simulink model "Signal_Builder_verif"  (Simulink 8.4)
settings: Solver=ode45  StartTime=0.0  StopTime=10.0  RelTol=1e-3
undefined symbols (not defined in the file): sigbuilder_block
settings Model: Creator=Romain  LastModifiedBy=hbourbou
settings DataIOCC: SignalLoggingSaveFormat=Dataset
settings OptimizationCC: ExpressionDepthLimit=128
settings DebuggingCC: SolverPrmCheckMsg=none  FcnCallInpInsideContextMsg=EnableAllAsError  FrameProcessingCompatibilityMsg=error  StateNameClashWarn=none
settings GRTTargetCC: CombineOutputUpdateFcns=on  GRTInterface=off

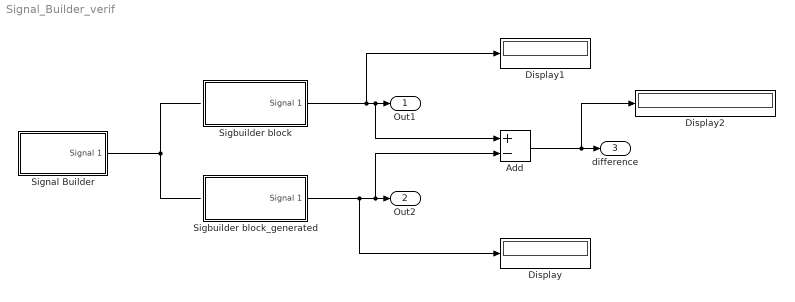
== system Signal_Builder_verif ==
  Add : Sum  Inputs=+-
  Display : Display
  Display1 : Display
  Display2 : Display
  Sigbuilder block : Subsystem  Tag=STV Subsys  LoadFcn=sigbuilder_block('load');  StartFcn=sigbuilder_block('start');  StopFcn=sigbuilder_block('stop');  ClipboardFcn=sigbuilder_block('clipboard');  mask(Sigbuilder block){}
      mask help: Simulink:masks:SigbuilderBlock_MD
      mask init:
      | if ~strcmp(get_param(bdroot(gcbh),'SimulationStatus'),'stopped') tuvar = sigbuilder_block('maskInit'); end
      settings: CopyFcn=sigbuilder_block('copy');  DeleteFcn=sigbuilder_block('delete');  ModelCloseFcn=sigbuilder_block('modelClose');  PreSaveFcn=sigbuilder_block('preSave');  PauseFcn=sigbuilder_block('pause');  ContinueFcn=sigbuilder_block('continue');  NameChangeFcn=sigbuilder_block('namechange');  OpenFcn=sigbuilder_block('open',[437.6 199.2 550.4 400 ]);  CloseFcn=sigbuilder_block('close');
      mask Display: plot(0, 0, 100, 100,[2, 2, 32, 32, 2], [68, 8, 8, 68, 68],[32, 2], [38, 38], [32, 19, 2],[53, 60, 44], [32, 17, 17, 2],[16, 16, 31, 31]);txt = getActiveGroup(gcbh);text(2, 100, txt,'verticalAlignment', 'top');
  Sigbuilder block_generated : Subsystem  TreatAsAtomicUnit=on
  Signal Builder : Subsystem  Tag=STV Subsys  LoadFcn=sigbuilder_block('load');  StartFcn=sigbuilder_block('start');  StopFcn=sigbuilder_block('stop');  ClipboardFcn=sigbuilder_block('clipboard');  mask(Sigbuilder block){}
      mask help: Simulink:masks:SigbuilderBlock_MD
      mask init:
      | if ~strcmp(get_param(bdroot(gcbh),'SimulationStatus'),'stopped') tuvar = sigbuilder_block('maskInit'); end
      settings: CopyFcn=sigbuilder_block('copy');  DeleteFcn=sigbuilder_block('delete');  ModelCloseFcn=sigbuilder_block('modelClose');  PreSaveFcn=sigbuilder_block('preSave');  PauseFcn=sigbuilder_block('pause');  ContinueFcn=sigbuilder_block('continue');  NameChangeFcn=sigbuilder_block('namechange');  OpenFcn=sigbuilder_block('open',[437.6 199.2 550.4 400 ]);  CloseFcn=sigbuilder_block('close');
      mask Display: plot(0, 0, 100, 100,[2, 2, 32, 32, 2], [68, 8, 8, 68, 68],[32, 2], [38, 38], [32, 19, 2],[53, 60, 44], [32, 17, 17, 2],[16, 16, 31, 31]);txt = getActiveGroup(gcbh);text(2, 100, txt,'verticalAlignment', 'top');
  Out1 : Outport
  Out2 : Outport  Port=2
  difference : Outport  Port=3
  wires:
  Signal Builder/1(Signal 1) -> ?
  Sigbuilder block/1(Signal 1) -> Display1/1, Add/1, Out1/1
  Sigbuilder block_generated/1(Signal 1) -> Display/1, Add/2, Out2/1
  Add/1 -> Display2/1, difference/1

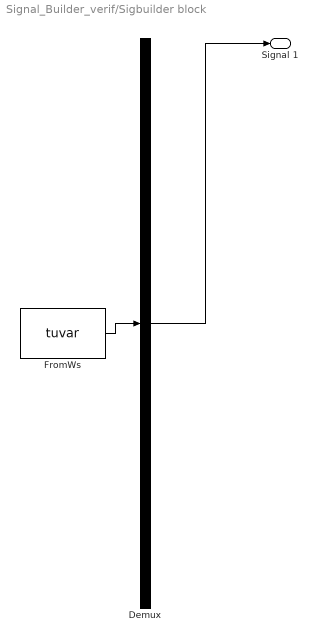
== system Signal_Builder_verif/Sigbuilder block ==
  Demux : Demux  Tag=STV Demux  Outputs=1
  FromWs : FromWorkspace  Tag=STV FromWs  VariableName=tuvar  SampleTime=0  SigBuilderData=DataTag0  VnvData=DataTag1
      SigBuilderData=|
      | common.afterFinalStr = 'Extrapolate'
      | common.sampleTime = 0
      | dataSet.timeRange = [0 10]
      | dataSet.name = 'Group 1'
      | sbobj.Groups.Name = 'Group 1'
      | sbobj.Groups.Signals.Name = 'Signal 1'
      | sbobj.Groups.Signals.XData = [0 4 4 6 6 10]
      | sbobj.Groups.Signals.YData = [0 0.99 1 0.01 0 0]
  Signal 1 : Outport  Tag=STV Outport
  wires:
  FromWs/1 -> Demux/1
  Demux/1 -> Signal 1/1

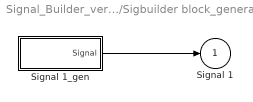
== system Signal_Builder_verif/Sigbuilder block_generated ==
  Signal 1_gen : Subsystem  TreatAsAtomicUnit=on
  Signal 1 : Outport
  wires:
  Signal 1_gen/1(Signal) -> Signal 1/1

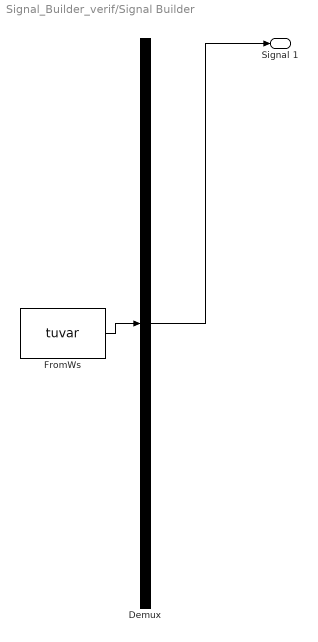
== system Signal_Builder_verif/Signal Builder ==
  Demux : Demux  Tag=STV Demux  Outputs=1
  FromWs : FromWorkspace  Tag=STV FromWs  VariableName=tuvar  SampleTime=0  SigBuilderData=DataTag2  VnvData=DataTag3
      SigBuilderData=|
      | common.afterFinalStr = 'Extrapolate'
      | common.sampleTime = 0
      | dataSet.timeRange = [0 10]
      | dataSet.name = 'Group 1'
      | sbobj.Groups.Name = 'Group 1'
      | sbobj.Groups.Signals.Name = 'Signal 1'
      | sbobj.Groups.Signals.XData = [0 4 4 6 6 10]
      | sbobj.Groups.Signals.YData = [0 0.99 1 0.3 0.26 0]
  Signal 1 : Outport  Tag=STV Outport
  wires:
  Demux/1 -> Signal 1/1
  FromWs/1 -> Demux/1

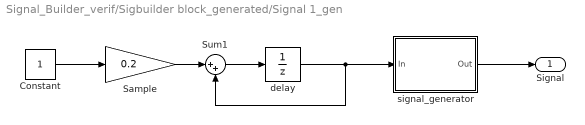
== system Signal_Builder_verif/Sigbuilder block_generated/Signal 1_gen ==
  Constant : Constant
  Sample : Gain  Gain=0.2
  Sum1 : Sum  RequirementInfo={} %GIDa_4fd8ee4a_06a5_4376_942d_ced6baffe973  Inputs=|++
  delay : UnitDelay  SampleTime=-1
  signal_generator : Subsystem  TreatAsAtomicUnit=on
  Signal : Outport  RequirementInfo={} %GIDa_242d5b11_f303_43fe_914a_b04d41914e6e
  wires:
  Sample/1 -> Sum1/1
  Sum1/1 -> delay/1
  Constant/1 -> Sample/1
  delay/1 -> Sum1/2, signal_generator/1(In)
  signal_generator/1(Out) -> Signal/1

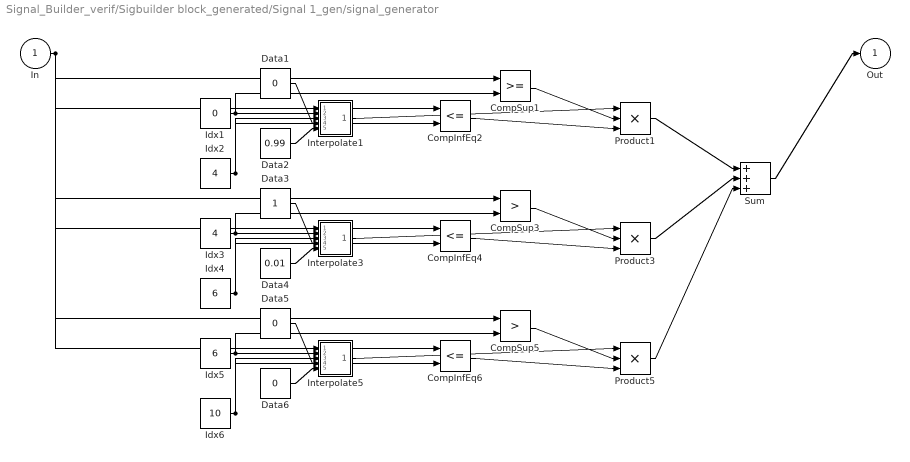
== system Signal_Builder_verif/Sigbuilder block_generated/Signal 1_gen/signal_generator ==
  In : Inport
  CompInfEq2 : RelationalOperator  Operator=<=  InputSameDT=on
  CompInfEq4 : RelationalOperator  Operator=<=  InputSameDT=on
  CompInfEq6 : RelationalOperator  Operator=<=  InputSameDT=on
  CompSup1 : RelationalOperator  InputSameDT=on
  CompSup3 : RelationalOperator  Operator=>  InputSameDT=on
  CompSup5 : RelationalOperator  Operator=>  InputSameDT=on
  Data1 : Constant  Value=0
  Data2 : Constant  Value=0.99
  Data3 : Constant
  Data4 : Constant  Value=0.01
  Data5 : Constant  Value=0
  Data6 : Constant  Value=0
  Idx1 : Constant  Value=0
  Idx2 : Constant  Value=4
  Idx3 : Constant  Value=4
  Idx4 : Constant  Value=6
  Idx5 : Constant  Value=6
  Idx6 : Constant  Value=10
  Interpolate1 : Subsystem  TreatAsAtomicUnit=on
  Interpolate3 : Subsystem  TreatAsAtomicUnit=on
  Interpolate5 : Subsystem  TreatAsAtomicUnit=on
  Product1 : Product  Inputs=***  SaturateOnIntegerOverflow=on  RndMeth=Zero  OutDataTypeStr=Inherit: Same as first input
  Product3 : Product  Inputs=***  SaturateOnIntegerOverflow=on  RndMeth=Zero  OutDataTypeStr=Inherit: Same as first input
  Product5 : Product  Inputs=***  SaturateOnIntegerOverflow=on  RndMeth=Zero  OutDataTypeStr=Inherit: Same as first input
  Sum : Sum  Inputs=+++  SaturateOnIntegerOverflow=on  InputSameDT=on  OutDataTypeStr=Inherit: Same as first input
  Out : Outport
  wires:
  Sum/1 -> Out/1
  Data6/1 -> Interpolate5/5(InportData2)
  Idx6/1 -> CompInfEq6/2, Interpolate5/3(InportIdx2)
  Product5/1 -> Sum/3
  CompInfEq6/1 -> Product5/3
  CompSup5/1 -> Product5/2
  Interpolate5/1(Out) -> Product5/1
  Data5/1 -> Interpolate5/4(InportData1)
  Idx5/1 -> CompSup5/2, Interpolate5/2(InportIdx1)
  Data4/1 -> Interpolate3/5(InportData2)
  Idx4/1 -> CompInfEq4/2, Interpolate3/3(InportIdx2)
  Product3/1 -> Sum/2
  CompInfEq4/1 -> Product3/3
  CompSup3/1 -> Product3/2
  Interpolate3/1(Out) -> Product3/1
  Data3/1 -> Interpolate3/4(InportData1)
  Idx3/1 -> CompSup3/2, Interpolate3/2(InportIdx1)
  Data2/1 -> Interpolate1/5(InportData2)
  Idx2/1 -> CompInfEq2/2, Interpolate1/3(InportIdx2)
  Product1/1 -> Sum/1
  CompInfEq2/1 -> Product1/3
  CompSup1/1 -> Product1/2
  Interpolate1/1(Out) -> Product1/1
  Data1/1 -> Interpolate1/4(InportData1)
  Idx1/1 -> CompSup1/2, Interpolate1/2(InportIdx1)
  In/1 -> CompInfEq6/1, CompSup5/1, Interpolate5/1(InportIn), CompInfEq4/1, CompSup3/1, Interpolate3/1(InportIn), CompInfEq2/1, CompSup1/1, Interpolate1/1(InportIn)

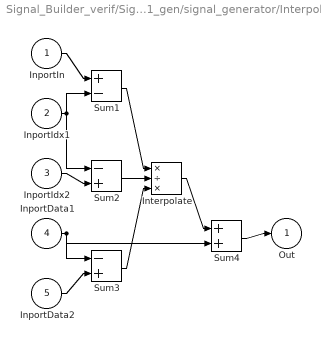
== system Signal_Builder_verif/Sigbuilder block_generated/Signal 1_gen/signal_generator/Interpolate1 ==
  InportIn : Inport
  InportIdx1 : Inport  Port=2
  InportIdx2 : Inport  Port=3
  InportData1 : Inport  Port=4
  InportData2 : Inport  Port=5
  Interpolate : Product  Inputs=*/*  SaturateOnIntegerOverflow=on  RndMeth=Zero  InputSameDT=on  OutDataTypeStr=Inherit: Same as first input
  Sum1 : Sum  Inputs=+-  SaturateOnIntegerOverflow=on  InputSameDT=on  OutDataTypeStr=Inherit: Same as first input
  Sum2 : Sum  Inputs=-+  SaturateOnIntegerOverflow=on  InputSameDT=on  OutDataTypeStr=Inherit: Same as first input
  Sum3 : Sum  Inputs=-+  SaturateOnIntegerOverflow=on  InputSameDT=on  OutDataTypeStr=Inherit: Same as first input
  Sum4 : Sum  SaturateOnIntegerOverflow=on  InputSameDT=on  OutDataTypeStr=Inherit: Same as first input
  Out : Outport
  wires:
  Sum4/1 -> Out/1
  Interpolate/1 -> Sum4/1
  Sum3/1 -> Interpolate/3
  Sum2/1 -> Interpolate/2
  Sum1/1 -> Interpolate/1
  InportData2/1 -> Sum3/2
  InportData1/1 -> Sum4/2, Sum3/1
  InportIdx2/1 -> Sum2/2
  InportIdx1/1 -> Sum2/1, Sum1/2
  InportIn/1 -> Sum1/1

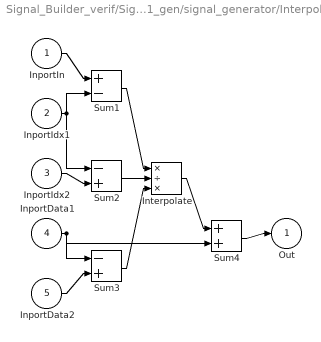
== system Signal_Builder_verif/Sigbuilder block_generated/Signal 1_gen/signal_generator/Interpolate3 ==
  InportIn : Inport
  InportIdx1 : Inport  Port=2
  InportIdx2 : Inport  Port=3
  InportData1 : Inport  Port=4
  InportData2 : Inport  Port=5
  Interpolate : Product  Inputs=*/*  SaturateOnIntegerOverflow=on  RndMeth=Zero  InputSameDT=on  OutDataTypeStr=Inherit: Same as first input
  Sum1 : Sum  Inputs=+-  SaturateOnIntegerOverflow=on  InputSameDT=on  OutDataTypeStr=Inherit: Same as first input
  Sum2 : Sum  Inputs=-+  SaturateOnIntegerOverflow=on  InputSameDT=on  OutDataTypeStr=Inherit: Same as first input
  Sum3 : Sum  Inputs=-+  SaturateOnIntegerOverflow=on  InputSameDT=on  OutDataTypeStr=Inherit: Same as first input
  Sum4 : Sum  SaturateOnIntegerOverflow=on  InputSameDT=on  OutDataTypeStr=Inherit: Same as first input
  Out : Outport
  wires:
  Sum4/1 -> Out/1
  Interpolate/1 -> Sum4/1
  Sum3/1 -> Interpolate/3
  Sum2/1 -> Interpolate/2
  Sum1/1 -> Interpolate/1
  InportData2/1 -> Sum3/2
  InportData1/1 -> Sum4/2, Sum3/1
  InportIdx2/1 -> Sum2/2
  InportIdx1/1 -> Sum2/1, Sum1/2
  InportIn/1 -> Sum1/1

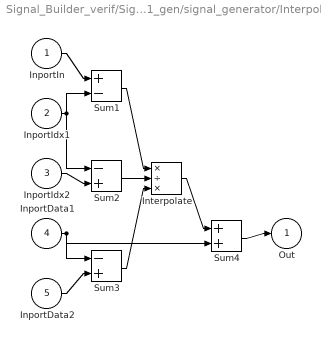
== system Signal_Builder_verif/Sigbuilder block_generated/Signal 1_gen/signal_generator/Interpolate5 ==
  InportIn : Inport
  InportIdx1 : Inport  Port=2
  InportIdx2 : Inport  Port=3
  InportData1 : Inport  Port=4
  InportData2 : Inport  Port=5
  Interpolate : Product  Inputs=*/*  SaturateOnIntegerOverflow=on  RndMeth=Zero  InputSameDT=on  OutDataTypeStr=Inherit: Same as first input
  Sum1 : Sum  Inputs=+-  SaturateOnIntegerOverflow=on  InputSameDT=on  OutDataTypeStr=Inherit: Same as first input
  Sum2 : Sum  Inputs=-+  SaturateOnIntegerOverflow=on  InputSameDT=on  OutDataTypeStr=Inherit: Same as first input
  Sum3 : Sum  Inputs=-+  SaturateOnIntegerOverflow=on  InputSameDT=on  OutDataTypeStr=Inherit: Same as first input
  Sum4 : Sum  SaturateOnIntegerOverflow=on  InputSameDT=on  OutDataTypeStr=Inherit: Same as first input
  Out : Outport
  wires:
  Sum4/1 -> Out/1
  Interpolate/1 -> Sum4/1
  Sum3/1 -> Interpolate/3
  Sum2/1 -> Interpolate/2
  Sum1/1 -> Interpolate/1
  InportData2/1 -> Sum3/2
  InportData1/1 -> Sum4/2, Sum3/1
  InportIdx2/1 -> Sum2/2
  InportIdx1/1 -> Sum2/1, Sum1/2
  InportIn/1 -> Sum1/1
